simulink model "Digital_modulation"  (R2021b)
settings: Solver=VariableStepAuto  StartTime=0.0  StopTime=1  MinStep=0.00001  RelTol=1e-3
libraries: commdigbbndpm3 x2, dspfdesign x2, commchan3 x1, commsink2 x1, commrandsrc3 x1
settings Model: Creator=user  LastModifiedBy=user

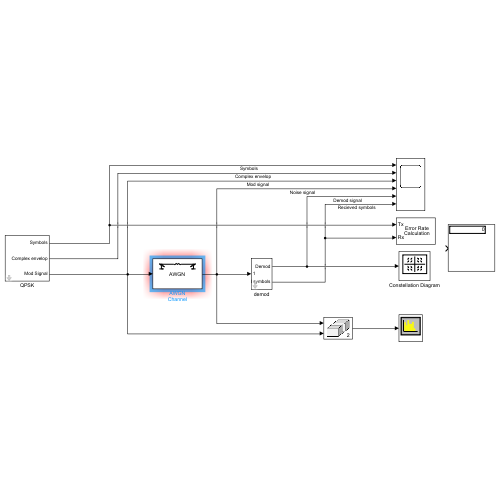
[thumbnail: Simulink's stored preview of the top-level diagram]
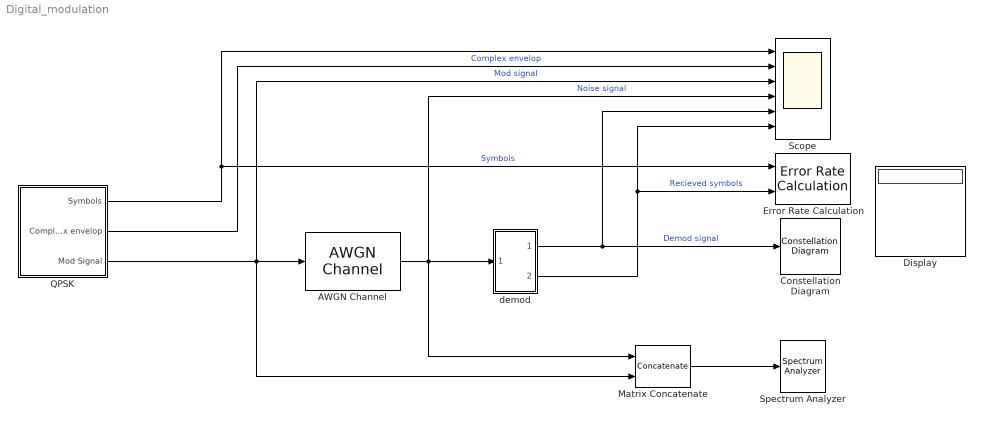
== system Digital_modulation ==
  AWGN Channel : commchan3/AWGN Channel  InputProcessing=Columns as channels (frame based)  seed=67  noiseMode="Signal to noise ratio  (SNR)"  EbNodB=EbNo  EsNodB=10  SNRdB=EbNo  bitsPerSym=1  Ps=1  Tsym=1  variance=1
  Constellation Diagram : ConstellationDiagram
  Display : Display
  Error Rate Calculation : commsink2/Error Rate Calculation  N=1  st_delay=0  cp_mode=Entire frame  subframe=[]  PMode=Workspace  WsName=ber  RsMode2=off  stop=off  numErr=100  maxBits=1e6
  Matrix Concatenate : Concatenate  Mode=Multidimensional array  ConcatenateDimension=2
  QPSK : Subsystem  mask{CarrierFrequency=1e4, SamplingFrequency=1e5, SymbolRate=1e3}
      mask prompts: CarrierFrequency "Carrier Frequency"; SamplingFrequency "Sampling Frequency"; SymbolRate "Symbol Rate"
  Scope : Scope  NumInputPorts=6
  Spectrum Analyzer : SpectrumAnalyzer
  demod : Subsystem  mask{CarrierFrequency=1e4, SymbolRate=1e3, SamplingFrequency=1e5}
      mask prompts: CarrierFrequency "Carrier Frequency"; SymbolRate "Symbol Rate"; SamplingFrequency "Sampling Frequency"
  wires:
  QPSK/3(Mod Signal) -> Matrix Concatenate/2, Scope/3, AWGN Channel/1  "Mod signal"
  AWGN Channel/1 -> Matrix Concatenate/1, Scope/4, demod/1(In1)  "Noise signal"
  QPSK/1(Symbols) -> Scope/1, Error Rate Calculation/1  "Symbols"
  QPSK/2(Complex envelop) -> Scope/2  "Complex envelop"
  demod/1(Demod) -> Constellation Diagram/1, Scope/5  "Demod signal"
  demod/2(Recieved symbols) -> Error Rate Calculation/2, Scope/6  "Recieved symbols"
  Matrix Concatenate/1 -> Spectrum Analyzer/1

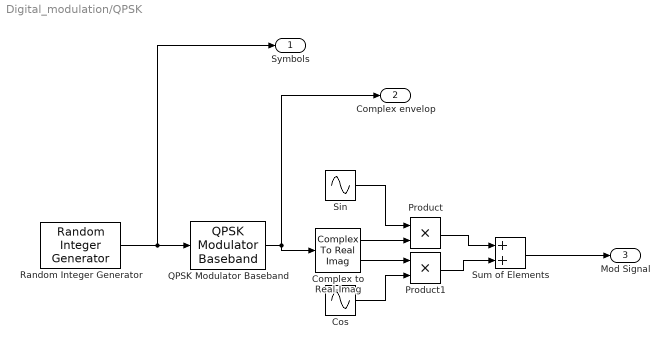
== system Digital_modulation/QPSK ==
  Complex to Real-Imag : ComplexToRealImag
  Cos : Sin  Frequency=2 * pi * CarrierFrequency  Phase=pi/2  SampleTime=1/SamplingFrequency
  Product : Product
  Product1 : Product
  QPSK Modulator Baseband : commdigbbndpm3/QPSK Modulator Baseband  InType=Integer  Enc=Gray  Ph=pi/4  outDtype=double  outWordLen=16  outUDDataType=sfix(16)  outFracLenMode=Best precision  outFracLen=15  outDataTypeStr=double  outLastDataTypeStr=double
  Random Integer Generator : commrandsrc3/Random Integer Generator  SetSize=4  SeedSource=Auto  Seed=0  SampleTime=1/SymbolRate  SamplesPerFrame=1  OutputDataType=uint8  SimulateUsing=Interpreted execution
  "Sin " : Sin  Frequency=2*pi*CarrierFrequency  SampleTime=1/SamplingFrequency
  Sum of Elements : Sum
  Symbols : Outport
  Complex envelop : Outport  Port=2
  Mod Signal : Outport  Port=3
  wires:
  Cos/1 -> Product1/2
  Complex to Real-Imag/2 -> Product1/1
  Product/1 -> Sum of Elements/1
  "Sin "/1 -> Product/1
  QPSK Modulator Baseband/1 -> Complex envelop/1, Complex to Real-Imag/1
  Product1/1 -> Sum of Elements/2
  Sum of Elements/1 -> Mod Signal/1
  Complex to Real-Imag/1 -> Product/2
  Random Integer Generator/1 -> Symbols/1, QPSK Modulator Baseband/1

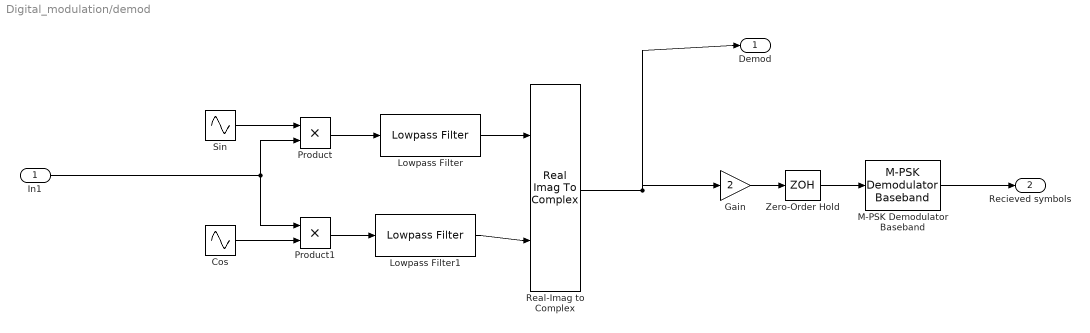
== system Digital_modulation/demod ==
  In1 : Inport
  Cos : Sin  Frequency=2 * pi * CarrierFrequency  Phase=pi / 2  SampleTime=1/SamplingFrequency
  Gain : Gain  Gain=2
  Lowpass Filter : dspfdesign/Lowpass Filter  FilterType=FIR  DesignForMinimumOrder=on  FilterOrder=50  PassbandFrequency=CarrierFrequency  StopbandFrequency=CarrierFrequency * 1.2  PassbandRipple=0.5  StopbandAttenuation=80  InheritSampleRate=on  SampleRate=SamplingFrequency  SimulateUsing=Interpreted execution  roundingMode=Floor  coeffsDataTypeStr=fixdt(1,16)
  Lowpass Filter1 : dspfdesign/Lowpass Filter  FilterType=FIR  DesignForMinimumOrder=on  FilterOrder=50  PassbandFrequency=CarrierFrequency  StopbandFrequency=CarrierFrequency * 1.2  PassbandRipple=0.5  StopbandAttenuation=80  InheritSampleRate=on  SampleRate=SamplingFrequency  SimulateUsing=Interpreted execution  roundingMode=Floor  coeffsDataTypeStr=fixdt(1,16)
  M-PSK Demodulator Baseband : commdigbbndpm3/M-PSK Demodulator Baseband  M=4  OutType=Integer  DecType=Hard decision  VarSource=Dialog  Variance=1  Dec=Gray  Mapping=[0:7]  Ph=pi/4  outDtype1=Inherit via internal rule  outDtype2=Inherit via internal rule  derotateFactorWordLen=16  derotateFactorDataTypeStr=Inherit: Same word length as input  derotateFactorLastDataTypeStr=Inherit: Same word length as input
  Product : Product
  Product1 : Product
  Real-Imag to Complex : RealImagToComplex
  "Sin " : Sin  Frequency=2 * pi * CarrierFrequency  SampleTime=1/SamplingFrequency
  Zero-Order Hold : ZeroOrderHold  SampleTime=1/SymbolRate
  Demod : Outport
  Recieved symbols : Outport  Port=2
  wires:
  Gain/1 -> Zero-Order Hold/1
  Product/1 -> Lowpass Filter/1
  In1/1 -> Product1/1, Product/2
  Real-Imag to Complex/1 -> Demod/1, Gain/1
  "Sin "/1 -> Product/1
  Product1/1 -> Lowpass Filter1/1
  Lowpass Filter1/1 -> Real-Imag to Complex/2
  Zero-Order Hold/1 -> M-PSK Demodulator Baseband/1
  Cos/1 -> Product1/2
  Lowpass Filter/1 -> Real-Imag to Complex/1
  M-PSK Demodulator Baseband/1 -> Recieved symbols/1
